simulink model "Model_C"  (R2021a)
settings: Solver=VariableStepAuto  StartTime=0.0  StopTime=10.0  RelTol=1e-3
values from neighbouring files (symbols this model uses):
  c1 = 100    [code_param.m]    (also in ode45_a.m; ode45_a1.m)
  c2 = 1000    [code_param.m]    (also in ode45_a.m; ode45_a1.m)
  k1 = 10^4    (= 10000)    [code_param.m]    (also in ode45_a.m; ode45_a1.m)
  k2 = 10^5    (= 100000)    [code_param.m]    (also in ode45_a.m; ode45_a1.m)
  m1 = 10    [code_param.m]    (also in ode45_a.m; ode45_a1.m)
  m2 = 100    [code_param.m]    (also in ode45_a.m; ode45_a1.m)
settings Model: Creator=Tushar  LastModifiedBy=Tushar

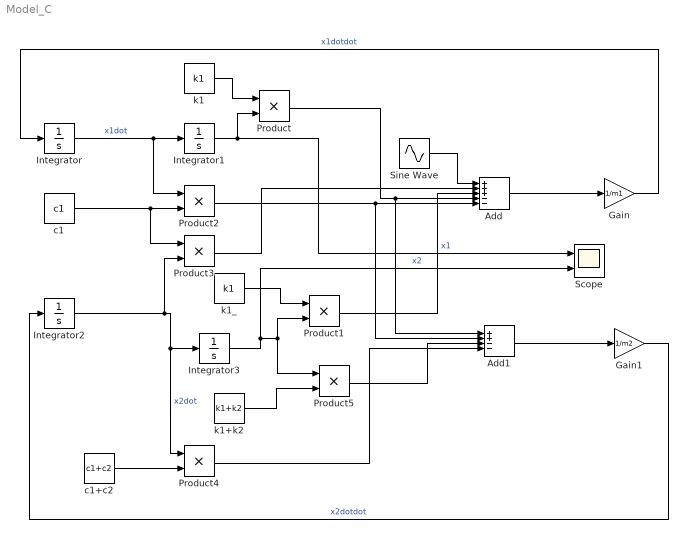
== system Model_C ==
  Add : Sum  Inputs=+++--
  Add1 : Sum  Inputs=++--
  Gain : Gain  Gain=1/m1
  Gain1 : Gain  Gain=1/m2
  Integrator{,1..3} (4 alike) : Integrator
  Product{,1..5} (6 alike) : Product
  Scope : Scope  NumInputPorts=2
  Sine Wave : Sin  Amplitude=3  Frequency=10  SampleTime=0
  c1 : Constant  Value=c1
  c1+c2 : Constant  Value=c1+c2
  k1 : Constant  Value=k1
  k1+k2 : Constant  Value=k1+k2
  k1_ : Constant  Value=k1
  wires:
  Product3/1 -> Add/2
  Product5/1 -> Add1/3
  Add/1 -> Gain/1
  c1/1 -> Product3/1, Product2/2
  Product/1 -> Add1/1, Add/4
  Product4/1 -> Add1/4
  Integrator3/1 -> Scope/2, Product5/1, Product1/2  "x2"
  k1/1 -> Product/1
  Sine Wave/1 -> Add/1
  k1_/1 -> Product1/1
  Add1/1 -> Gain1/1
  Product1/1 -> Add/3
  Integrator2/1 -> Product3/2, Product4/1, Integrator3/1  "x2dot"
  Integrator/1 -> Product2/1, Integrator1/1  "x1dot"
  Gain1/1 -> Integrator2/1  "x2dotdot"
  c1+c2/1 -> Product4/2
  k1+k2/1 -> Product5/2
  Product2/1 -> Add1/2, Add/5
  Integrator1/1 -> Scope/1, Product/2  "x1"
  Gain/1 -> Integrator/1  "x1dotdot"
